simulink model "connect_pend_add"  (R2019b)
settings: Solver=VariableStepAuto  StartTime=0.0  StopTime=10.0  RelTol=1e-3
values from neighbouring files (symbols this model uses):
  Bd = 50    [anujay_single_pendulum_same.m]    (also in connect_pend_runner.m; double_pend_setup.m = [50,0;0,50])
  dampener = 100    [anujay_single_pendulum_same.m]    (also in connect_pend.m; connect_pend_runner.m; double_pend_setup.m = [50, 0; 0, 50])
  Dm1 = 30    [anujay_single_pendulum_same.m]    (also in connect_pend.m; connect_pend_runner.m; double_pend_setup.m = [30,0;0,30])
  g = 9.81    [G.m]    (also in connect_pend_runner.m = -9.81; run.m; single_pend_runner.m = -9.81)
  Kd = 50    [anujay_single_pendulum_same.m]    (also in connect_pend_runner.m; double_pend_setup.m = [50,0;0,50]; run.m = 300; single_pend_runner.m = 500)
  Km1 = 30    [anujay_single_pendulum_same.m]    (also in connect_pend.m; connect_pend_runner.m; double_pend_setup.m = [30, 0; 0 30])
  l1 = 1.0    (= 1)    [connect_pend.m]    (also in connect_pend_runner.m)
  l2 = l1    (= 1)    [connect_pend_runner.m]    (also in single_pend_runner.m = 3)
  lambda = 50.0    (= 50)    [connect_pend_runner.m]    (also in single_pend_runner.m = 1)
  lambda2 = 1.2    [anujay_single_pendulum_same.m]    (also in connect_pend_runner.m = 2.8; double_pend_setup.m = [5.0, 0; 0 5.0])
  m1 = 1.0    (= 1)    [connect_pend.m]    (also in connect_pend_runner.m)
  m2 = 1.0 + m1    (= 2)    [connect_pend.m]    (also in connect_pend_runner.m; single_pend_runner.m = 10)
  Md = 10    [anujay_single_pendulum_same.m]    (also in connect_pend_runner.m; double_pend_setup.m = [10, 0; 0, 20])
  rho = .50    (= 0.5)    [connect_pend_runner.m]
  rho2 = 100    [anujay_single_pendulum_same.m]    (also in connect_pend_runner.m = 4.5; double_pend_setup.m = [18, 0; 0, 18])
  spring = 100    [anujay_single_pendulum_same.m]    (also in connect_pend.m; connect_pend_runner.m; double_pend_setup.m = [50, 0; 0, 50])
libraries: robotcorelib x3, simulink x2
settings Model: Creator=nathanielgoldfarb  LastModifiedBy=nathanielgoldfarb
settings SolverCC: ZeroCrossAlgorithm=Adaptive
settings DebuggingCC: IgnoredZcDiagnostic=none

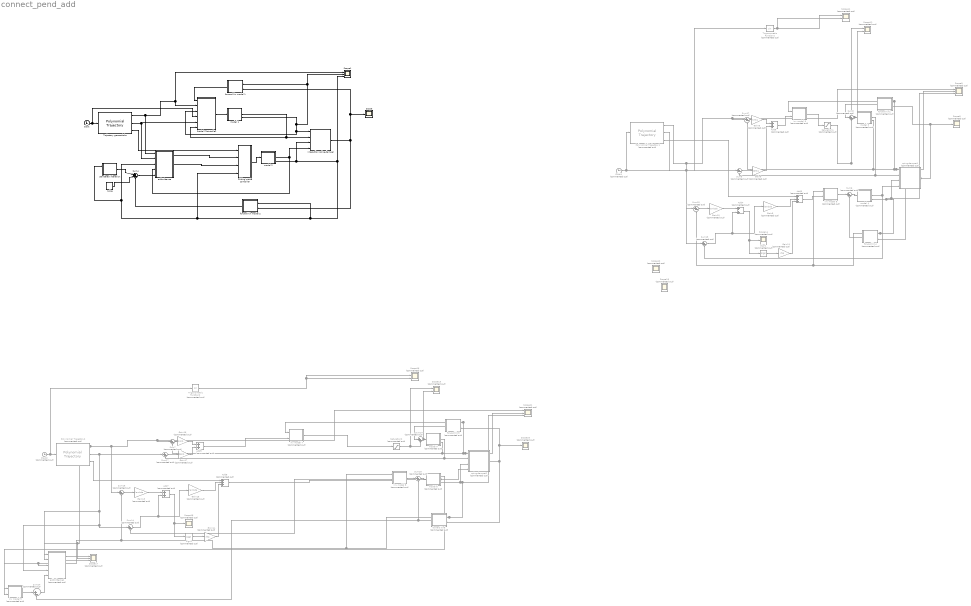
== system connect_pend_add ==
  " interaction sping-damper" : Subsystem
  Add{4,6..7,9} (4 alike) : Sum  Commented=on
  Add5 : Sum  Commented=on  Inputs=+++
  Add8 : Sum  Commented=on  Inputs=+++
  Clock : Clock
  Clock1 : Clock  Commented=on
  Clock2 : Clock  Commented=on
  Gain{5,10,13,15} (4 alike) : Gain  Commented=on  Gain=lambda
  Gain11 : Gain  Commented=on  Gain=rho
  Gain14 : Gain  Commented=on  Gain=rho
  Gain16 : Gain  Commented=on  Gain=Km1
  Gain17 : Gain  Commented=on  Gain=Dm1
  Gain8 : Gain  Commented=on  Gain=Km1
  Gain9 : Gain  Commented=on  Gain=Dm1
  Polynomial Trajectory1 : robotcorelib/Polynomial Trajectory  Commented=on  WaypointSource=Internal  Waypoints=[ -pi , 0 ]  TimePoints=[ 0, 3]  TimeInterval=[ 1, 4 ]  Method=Cubic Polynomial  ParameterSource=Internal  VelocityBoundaryCondition=zeros( 1, 2 )  AccelerationBoundaryCondition=zeros( 2, 5 )  SimulateUsing=Interpreted execution
      settings: SourceProductName=Robotics System Toolbox  SourceProductBaseCode=RO
  Polynomial Trajectory2 : robotcorelib/Polynomial Trajectory  Commented=on  WaypointSource=Internal  Waypoints=[ -pi , 0 ]  TimePoints=[ 0, 3]  TimeInterval=[ 1, 4 ]  Method=Cubic Polynomial  ParameterSource=Internal  VelocityBoundaryCondition=zeros( 1, 2 )  AccelerationBoundaryCondition=zeros( 2, 5 )  SimulateUsing=Interpreted execution
      settings: SourceProductName=Robotics System Toolbox  SourceProductBaseCode=RO
  Saturation1 : Saturate  Commented=on  UpperLimit=1.0  LowerLimit=-1.0
  Saturation2 : Saturate  Commented=on  UpperLimit=1.0  LowerLimit=-1.0
  Scope : Scope
  Scope1 : Scope  NumInputPorts=3
  Scope{10..13,15..16} (6 alike) : Scope  Commented=on  NumInputPorts=2
  Scope{8,14,18,20} (4 alike) : Scope  Commented=on
  Scope17 : Scope  Commented=on  NumInputPorts=3
  Scope21 : Scope  Commented=on  NumInputPorts=3
  Scope9 : Scope  Commented=on  NumInputPorts=3
  Sign1 : Signum  Commented=on
  Sign2 : Signum  Commented=on
  Sum{5..7,12..18,20} (11 alike) : Sum  Commented=on  Inputs=|+-
  Sum19 : Sum  Commented=on  Inputs=|++
  Sum4 : Sum  Inputs=|++-
  Sum8 : Sum  Commented=on  Inputs=|++
  Trajectory generatiobn : robotcorelib/Polynomial Trajectory  WaypointSource=Internal  Waypoints=[ -pi , 0 ]  TimePoints=[ 0, 3]  TimeInterval=[ 1, 4 ]  Method=Cubic Polynomial  ParameterSource=Internal  VelocityBoundaryCondition=zeros( 1, 2 )  AccelerationBoundaryCondition=zeros( 2, 5 )  SimulateUsing=Interpreted execution
      settings: SourceProductName=Robotics System Toolbox  SourceProductBaseCode=RO
  Trigonometric Function1 : Trigonometry  Commented=on
  Trigonometric Function2 : Trigonometry  Commented=on
  addmittacne1 : Subsystem  Commented=on
  addmittance : Subsystem
  forward kin model 1 : Subsystem
  forward kin model 2 : Subsystem
  forward kin1 : Subsystem  Commented=on
  forward kin4 : Subsystem  Commented=on
  forward kin5 : Subsystem  Commented=on
  forward kin6 : Subsystem  Commented=on
  inv model 5 : Subsystem  Commented=on
  inv model 6 : Subsystem  Commented=on
  inv model 7 : Subsystem  Commented=on
  inv model 8 : Subsystem  Commented=on
  inv model 9 : Subsystem  Commented=on
  model 1 : Subsystem
  model 1 controller : Subsystem
  model 2 : Subsystem
  model 3 : Subsystem  Commented=on
  model 4 : Subsystem  Commented=on
  model 5 : Subsystem  Commented=on
  model 6 : Subsystem  Commented=on
  noise : UniformRandomNumber  Minimum=-3  Maximum=3  SampleTime=0.1
  sliding mode controller : Subsystem
  sping-damper1 : Subsystem  Commented=on
  sping-damper2 : Subsystem  Commented=on
  standered interation : Subsystem
  wires:
  model 1/3(pos) -> model 1 controller/3(q), " interaction sping-damper"/1(theta 1), Scope1/2, forward kin model 1/1("theta ")  "model 1"
  " interaction sping-damper"/1(F) -> Scope/1, forward kin model 1/2(F), forward kin model 2/2(F)
  model 2/3(pos) -> forward kin model 2/1("theta "), addmittance/3(q), standered interation/1(q), sliding mode controller/4(q), Scope1/3, " interaction sping-damper"/3(theta 2)  "model 2"
  model 2/2(vel) -> addmittance/4(qd), " interaction sping-damper"/4(dtheta 2)  "model 2"
  forward kin model 2/1("tau ") -> Sum4/3  "Ti"
  Sum4/1 -> addmittance/5(force)
  standered interation/1("tau ") -> Sum4/1  "Tid"
  model 4/3(pos) -> Scope9/3, sping-damper1/3(theta 2), Sum15/2, inv model 6/1(q), forward kin4/1("theta ")  "model 2"
  sping-damper1/1(F) -> Scope8/1, forward kin1/2(F), forward kin4/2(F)
  Add6/1 -> inv model 5/2("u ")
  Clock1/1 -> Trigonometric Function1/1, Polynomial Trajectory1/1
  model 3/3(pos) -> forward kin1/1("theta "), inv model 5/1(q), Scope9/2, sping-damper1/1(theta 1), Sum12/2  "model 1"
  Gain11/1 -> Add5/3
  Gain10/1 -> Add4/1
  forward kin1/1("tau ") -> Sum8/1
  Add5/1 -> inv model 6/2("u ")
  Gain9/1 -> Add6/2
  Saturation1/1 -> Scope10/1, Sum8/2
  model 4/2(vel) -> sping-damper1/4(dtheta 2), Sum13/2  "model 2"
  Sum12/1 -> Gain8/1
  Sign1/1 -> Gain11/1
  Trigonometric Function1/1 -> Scope11/1, Scope11/2
  inv model 5/1("tau ") -> Saturation1/1
  model 3/2(vel) -> sping-damper1/2(dtheta 1), Sum5/2
  Gain8/1 -> Add6/1
  Sum8/1 -> Scope10/2, model 3/1("u ")
  Sum5/1 -> Gain9/1
  Add4/1 -> Sign1/1, Scope14/1
  Polynomial Trajectory1/2 -> Sum5/1, Sum13/1
  Polynomial Trajectory1/1 -> Scope9/1, Sum12/1, Sum15/1
  Sum15/1 -> Gain10/1
  Sum13/1 -> Gain5/1, Add4/2
  Polynomial Trajectory1/3 -> Add5/1
  inv model 6/1("tau ") -> Sum6/1  "SMC"
  Sum6/1 -> model 4/1("u ")
  Gain5/1 -> Add5/2
  forward kin4/1("tau ") -> Sum6/2
  Gain13/1 -> Add7/1
  Gain14/1 -> Add8/3
  Gain17/1 -> Add9/2
  Add8/1 -> inv model 8/2("u ")
  Sum14/1 -> Gain15/1, Add7/2
  model 5/2(vel) -> sping-damper2/2(dtheta 1), Sum17/2
  Sum17/1 -> Gain17/1
  Add9/1 -> inv model 7/2("u ")
  Sign2/1 -> Gain14/1
  Clock2/1 -> Trigonometric Function2/1, Polynomial Trajectory2/1
  sping-damper2/1(F) -> forward kin6/2(F), Scope20/1, forward kin5/2(F)
  Sum19/1 -> Scope13/2, model 5/1("u ")
  Gain15/1 -> Add8/2
  Saturation2/1 -> Scope13/1, Sum19/2
  Polynomial Trajectory2/1 -> Scope21/1, Sum7/1, Sum16/1, addmittacne1/1(q desird), Scope17/2
  inv model 8/1("tau ") -> Sum18/1  "SMC"
  Sum7/1 -> Gain16/1
  forward kin6/1("tau ") -> Sum20/2, Sum18/2
  model 6/3(pos) -> Scope21/3, inv model 9/1(q), addmittacne1/3(q), Scope17/3, Sum16/2, inv model 8/1(q), forward kin6/1("theta "), sping-damper2/3(theta 2)  "model 2"
  Polynomial Trajectory2/3 -> Add8/1
  forward kin5/1("tau ") -> Sum19/1
  model 5/3(pos) -> forward kin5/1("theta "), inv model 7/1(q), Scope21/2, sping-damper2/1(theta 1), Sum7/2  "model 1"
  Sum16/1 -> Gain13/1
  Polynomial Trajectory2/2 -> Sum17/1, addmittacne1/2(qd desird), Sum14/1, addmittacne1/4(qd)
  model 6/2(vel) -> sping-damper2/4(dtheta 2), Sum14/2  "model 2"
  inv model 7/1("tau ") -> Saturation2/1
  Sum18/1 -> model 6/1("u ")
  Gain16/1 -> Add9/1
  Add7/1 -> Sign2/1, Scope18/1
  Trigonometric Function2/1 -> Scope16/1, Scope16/2
  inv model 9/1("tau ") -> Sum20/1  "SMC"
  Sum20/1 -> addmittacne1/5(force)
  model 6/1(accel) -> inv model 9/2("u ")
  addmittacne1/1(q_add) -> Scope17/1
  noise/1 -> Sum4/2
  addmittance/1(q_add) -> sliding mode controller/2(x)  "x"
  model 1/2(vel) -> model 1 controller/6(qd), " interaction sping-damper"/2(dtheta 1)
  Trajectory generatiobn/2 -> model 1 controller/5(qd desired), addmittance/2(qd desird)
  Trajectory generatiobn/1 -> addmittance/1(q desird), model 1 controller/2(q desired), Scope1/1
  Clock/1 -> model 1 controller/4(t), Trajectory generatiobn/1
  forward kin model 1/1("tau ") -> model 1 controller/1(interaction torque)
  model 1 controller/1(u) -> model 1/1("u ")
  Trajectory generatiobn/3 -> sliding mode controller/1(qdd desired)
  addmittance/2(qd_add) -> sliding mode controller/3(xd)  "xd"
  sliding mode controller/1(SMC) -> model 2/1("u ")

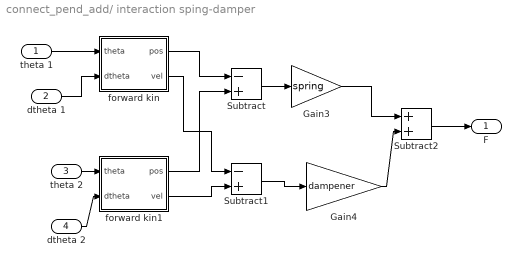
== system connect_pend_add/ interaction sping-damper ==
  theta 1 : Inport
  dtheta 1 : Inport  Port=2
  theta 2 : Inport  Port=3
  dtheta 2 : Inport  Port=4
  Gain3 : Gain  Gain=spring
  Gain4 : Gain  Gain=dampener
  Subtract : Sum  Inputs=-+
  Subtract1 : Sum  Inputs=-+
  Subtract2 : Sum
  forward kin : Subsystem
  forward kin1 : Subsystem
  F : Outport
  wires:
  Subtract2/1 -> F/1
  forward kin/2(vel) -> Subtract1/1
  Gain4/1 -> Subtract2/2
  Subtract1/1 -> Gain4/1
  dtheta 1/1 -> forward kin/2("dtheta ")
  forward kin1/1(pos) -> Subtract/2
  theta 1/1 -> forward kin/1("theta ")
  Subtract/1 -> Gain3/1
  forward kin/1(pos) -> Subtract/1
  dtheta 2/1 -> forward kin1/2("dtheta ")
  theta 2/1 -> forward kin1/1("theta ")
  forward kin1/2(vel) -> Subtract1/2
  Gain3/1 -> Subtract2/1

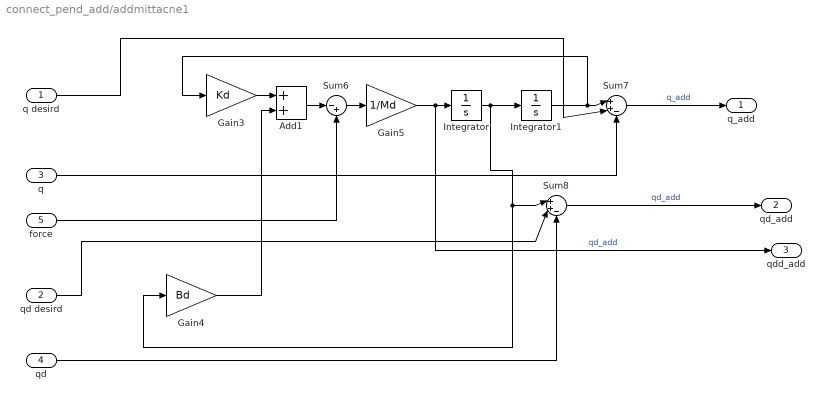
== system connect_pend_add/addmittacne1 ==
  q desird : Inport
  qd desird : Inport  Port=2
  q : Inport  Port=3
  qd : Inport  Port=4
  force : Inport  Port=5
  Add1 : Sum
  Gain3 : Gain  Gain=Kd
  Gain4 : Gain  Gain=Bd
  Gain5 : Gain  Gain=1/Md
  Integrator : Integrator
  Integrator1 : Integrator  InitialCondition=-3
  Sum6 : Sum  Inputs=|-+
  Sum7 : Sum  Inputs=|++-
  Sum8 : Sum  Inputs=|++-
  q_add : Outport
  qd_add : Outport  Port=2
  qdd_add : Outport  Port=3
  wires:
  Sum6/1 -> Gain5/1
  Integrator1/1 -> Gain3/1, Sum7/1
  Integrator/1 -> Gain4/1, Sum8/1, Integrator1/1
  q desird/1 -> Sum7/2
  Gain3/1 -> Add1/1
  Gain4/1 -> Add1/2
  force/1 -> Sum6/2
  qd desird/1 -> Sum8/2
  Sum8/1 -> qd_add/1  "qd_add"
  Add1/1 -> Sum6/1
  Sum7/1 -> q_add/1  "q_add"
  Gain5/1 -> qdd_add/1, Integrator/1  "qd_add"
  qd/1 -> Sum8/3
  q/1 -> Sum7/3

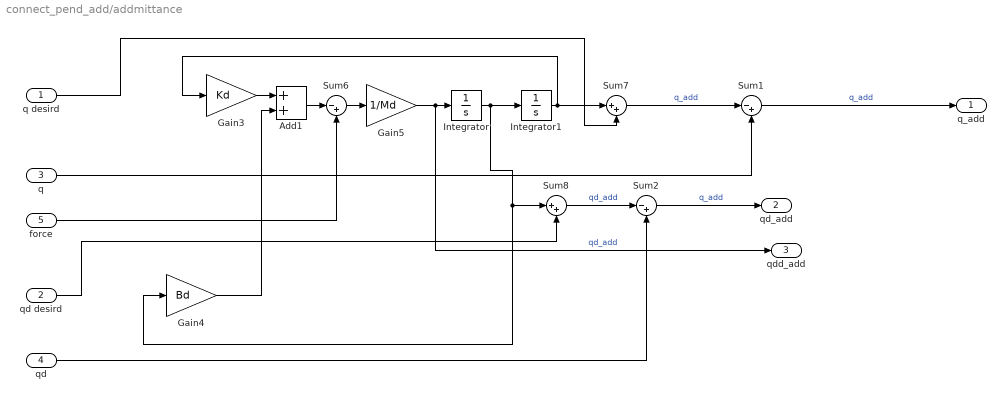
== system connect_pend_add/addmittance ==
  q desird : Inport
  qd desird : Inport  Port=2
  q : Inport  Port=3
  qd : Inport  Port=4
  force : Inport  Port=5
  Add1 : Sum
  Gain3 : Gain  Gain=Kd
  Gain4 : Gain  Gain=Bd
  Gain5 : Gain  Gain=1/Md
  Integrator : Integrator
  Integrator1 : Integrator  InitialCondition=pi
  Sum1 : Sum  Inputs=|-+
  Sum2 : Sum  Inputs=|-+
  Sum6 : Sum  Inputs=|-+
  Sum7 : Sum  Inputs=|++
  Sum8 : Sum  Inputs=|++
  q_add : Outport
  qd_add : Outport  Port=2
  qdd_add : Outport  Port=3
  wires:
  Sum7/1 -> Sum1/1  "q_add"
  Add1/1 -> Sum6/1
  force/1 -> Sum6/2
  qd desird/1 -> Sum8/2
  Gain5/1 -> qdd_add/1, Integrator/1  "qd_add"
  Sum6/1 -> Gain5/1
  Gain4/1 -> Add1/2
  Gain3/1 -> Add1/1
  Integrator/1 -> Gain4/1, Sum8/1, Integrator1/1
  q desird/1 -> Sum7/2
  Sum8/1 -> Sum2/1  "qd_add"
  Integrator1/1 -> Gain3/1, Sum7/1
  qd/1 -> Sum2/2
  Sum1/1 -> q_add/1  "q_add"
  q/1 -> Sum1/2
  Sum2/1 -> qd_add/1  "q_add"

== system connect_pend_add/forward kin model 1 ==
  "theta " : Inport
  F : Inport  Port=2
  Gain3 : Gain  Gain=-l1
  Gain4 : Gain  Gain=l1
  Mux : Mux  Inputs=2
  Product : Product  Multiplication=Matrix(*)
  Transpose : Math  Operator=transpose  SignedPower=off  SaturateOnIntegerOverflow=on
  Trigonometric Function : Trigonometry
  Trigonometric Function1 : Trigonometry  Operator=cos
  XY Graph : simulink/Sinks/XY Graph  xmin=-1  xmax=1  ymin=-1  ymax=1  st=-1
  "tau " : Outport
  wires:
  "theta "/1 -> Trigonometric Function1/1, Trigonometric Function/1
  Gain4/1 -> XY Graph/2, Mux/2
  Trigonometric Function/1 -> Gain3/1
  Gain3/1 -> XY Graph/1, Mux/1
  Trigonometric Function1/1 -> Gain4/1
  Mux/1 -> Transpose/1
  Transpose/1 -> Product/1
  F/1 -> Product/2
  Product/1 -> "tau "/1

== system connect_pend_add/forward kin model 2 ==
  "theta " : Inport
  F : Inport  Port=2
  Gain3 : Gain  Gain=-l1
  Gain4 : Gain  Gain=l1
  Mux : Mux  Inputs=2
  Product : Product  Multiplication=Matrix(*)
  Transpose : Math  Operator=transpose  SignedPower=off  SaturateOnIntegerOverflow=on
  Trigonometric Function : Trigonometry
  Trigonometric Function1 : Trigonometry  Operator=cos
  "tau " : Outport
  wires:
  "theta "/1 -> Trigonometric Function1/1, Trigonometric Function/1
  Gain4/1 -> Mux/2
  Trigonometric Function/1 -> Gain3/1
  Gain3/1 -> Mux/1
  Trigonometric Function1/1 -> Gain4/1
  Mux/1 -> Transpose/1
  Transpose/1 -> Product/1
  F/1 -> Product/2
  Product/1 -> "tau "/1

== system connect_pend_add/forward kin1 ==
  "theta " : Inport
  F : Inport  Port=2
  Gain3 : Gain  Gain=-l1
  Gain4 : Gain  Gain=l1
  Mux : Mux  Inputs=2
  Product : Product  Multiplication=Matrix(*)
  Transpose : Math  Operator=transpose  SignedPower=off  SaturateOnIntegerOverflow=on
  Trigonometric Function : Trigonometry
  Trigonometric Function1 : Trigonometry  Operator=cos
  "tau " : Outport
  wires:
  "theta "/1 -> Trigonometric Function1/1, Trigonometric Function/1
  Gain4/1 -> Mux/2
  Trigonometric Function/1 -> Gain3/1
  Gain3/1 -> Mux/1
  Trigonometric Function1/1 -> Gain4/1
  Mux/1 -> Transpose/1
  Transpose/1 -> Product/1
  F/1 -> Product/2
  Product/1 -> "tau "/1

== system connect_pend_add/forward kin4 ==
  "theta " : Inport
  F : Inport  Port=2
  Gain3 : Gain  Gain=-l1
  Gain4 : Gain  Gain=l1
  Mux : Mux  Inputs=2
  Product : Product  Multiplication=Matrix(*)
  Transpose : Math  Operator=transpose  SignedPower=off  SaturateOnIntegerOverflow=on
  Trigonometric Function : Trigonometry
  Trigonometric Function1 : Trigonometry  Operator=cos
  "tau " : Outport
  wires:
  "theta "/1 -> Trigonometric Function1/1, Trigonometric Function/1
  Gain4/1 -> Mux/2
  Trigonometric Function/1 -> Gain3/1
  Gain3/1 -> Mux/1
  Trigonometric Function1/1 -> Gain4/1
  Mux/1 -> Transpose/1
  Transpose/1 -> Product/1
  F/1 -> Product/2
  Product/1 -> "tau "/1

== system connect_pend_add/forward kin5 ==
  "theta " : Inport
  F : Inport  Port=2
  Gain3 : Gain  Gain=-l1
  Gain4 : Gain  Gain=l1
  Mux : Mux  Inputs=2
  Product : Product  Multiplication=Matrix(*)
  Transpose : Math  Operator=transpose  SignedPower=off  SaturateOnIntegerOverflow=on
  Trigonometric Function : Trigonometry
  Trigonometric Function1 : Trigonometry  Operator=cos
  "tau " : Outport
  wires:
  "theta "/1 -> Trigonometric Function1/1, Trigonometric Function/1
  Gain4/1 -> Mux/2
  Trigonometric Function/1 -> Gain3/1
  Gain3/1 -> Mux/1
  Trigonometric Function1/1 -> Gain4/1
  Mux/1 -> Transpose/1
  Transpose/1 -> Product/1
  F/1 -> Product/2
  Product/1 -> "tau "/1

== system connect_pend_add/forward kin6 ==
  "theta " : Inport
  F : Inport  Port=2
  Gain3 : Gain  Gain=-l1
  Gain4 : Gain  Gain=l1
  Mux : Mux  Inputs=2
  Product : Product  Multiplication=Matrix(*)
  Transpose : Math  Operator=transpose  SignedPower=off  SaturateOnIntegerOverflow=on
  Trigonometric Function : Trigonometry
  Trigonometric Function1 : Trigonometry  Operator=cos
  "tau " : Outport
  wires:
  "theta "/1 -> Trigonometric Function1/1, Trigonometric Function/1
  Gain4/1 -> Mux/2
  Trigonometric Function/1 -> Gain3/1
  Gain3/1 -> Mux/1
  Trigonometric Function1/1 -> Gain4/1
  Mux/1 -> Transpose/1
  Transpose/1 -> Product/1
  F/1 -> Product/2
  Product/1 -> "tau "/1

== system connect_pend_add/inv model 5 ==
  q : Inport
  "u " : Inport  Port=2
  Add1 : Sum
  Constant1 : Constant  Value=m1*g*l1
  Gain3 : Gain  Gain=m1*l1*l1
  Product1 : Product
  Trigonometric Function1 : Trigonometry
  "tau " : Outport
  wires:
  Product1/1 -> Add1/1
  Constant1/1 -> Product1/2
  Add1/1 -> "tau "/1
  Gain3/1 -> Add1/2
  "u "/1 -> Gain3/1
  Trigonometric Function1/1 -> Product1/1
  q/1 -> Trigonometric Function1/1

== system connect_pend_add/inv model 6 ==
  q : Inport
  "u " : Inport  Port=2
  Add1 : Sum
  Constant1 : Constant  Value=m2*g*l2
  Gain3 : Gain  Gain=m2*l2*l2
  Product1 : Product
  Trigonometric Function1 : Trigonometry
  "tau " : Outport
  wires:
  Product1/1 -> Add1/1
  Constant1/1 -> Product1/2
  Add1/1 -> "tau "/1
  Gain3/1 -> Add1/2
  "u "/1 -> Gain3/1
  Trigonometric Function1/1 -> Product1/1
  q/1 -> Trigonometric Function1/1

== system connect_pend_add/inv model 7 ==
  q : Inport
  "u " : Inport  Port=2
  Add1 : Sum
  Constant1 : Constant  Value=m1*g*l1
  Gain3 : Gain  Gain=m1*l1*l1
  Product1 : Product
  Trigonometric Function1 : Trigonometry
  "tau " : Outport
  wires:
  Product1/1 -> Add1/1
  Constant1/1 -> Product1/2
  Add1/1 -> "tau "/1
  Gain3/1 -> Add1/2
  "u "/1 -> Gain3/1
  Trigonometric Function1/1 -> Product1/1
  q/1 -> Trigonometric Function1/1

== system connect_pend_add/inv model 8 ==
  q : Inport
  "u " : Inport  Port=2
  Add1 : Sum
  Constant1 : Constant  Value=m2*g*l2
  Gain3 : Gain  Gain=m2*l2*l2
  Product1 : Product
  Trigonometric Function1 : Trigonometry
  "tau " : Outport
  wires:
  Product1/1 -> Add1/1
  Constant1/1 -> Product1/2
  Add1/1 -> "tau "/1
  Gain3/1 -> Add1/2
  "u "/1 -> Gain3/1
  Trigonometric Function1/1 -> Product1/1
  q/1 -> Trigonometric Function1/1

== system connect_pend_add/inv model 9 ==
  q : Inport
  "u " : Inport  Port=2
  Add1 : Sum
  Constant1 : Constant  Value=m2*g*l2
  Gain3 : Gain  Gain=m2*l2*l2
  Product1 : Product
  Trigonometric Function1 : Trigonometry
  "tau " : Outport
  wires:
  Product1/1 -> Add1/1
  Constant1/1 -> Product1/2
  Add1/1 -> "tau "/1
  Gain3/1 -> Add1/2
  "u "/1 -> Gain3/1
  Trigonometric Function1/1 -> Product1/1
  q/1 -> Trigonometric Function1/1

== system connect_pend_add/model 1 ==
  "u " : Inport
  Add : Sum  Inputs=+-
  Constant : Constant  Value=m1*g*l1
  Gain : Gain  Gain=1/(m1*l1*l1)
  Integrator : Integrator
  Integrator1 : Integrator  InitialCondition=-pi
  Product : Product
  Trigonometric Function : Trigonometry
  accel : Outport
  vel : Outport  Port=2
  pos : Outport  Port=3
  wires:
  Integrator1/1 -> pos/1, Trigonometric Function/1
  "u "/1 -> Add/1
  Constant/1 -> Product/2
  Add/1 -> Gain/1
  Trigonometric Function/1 -> Product/1
  Product/1 -> Add/2
  Gain/1 -> accel/1, Integrator/1
  Integrator/1 -> vel/1, Integrator1/1

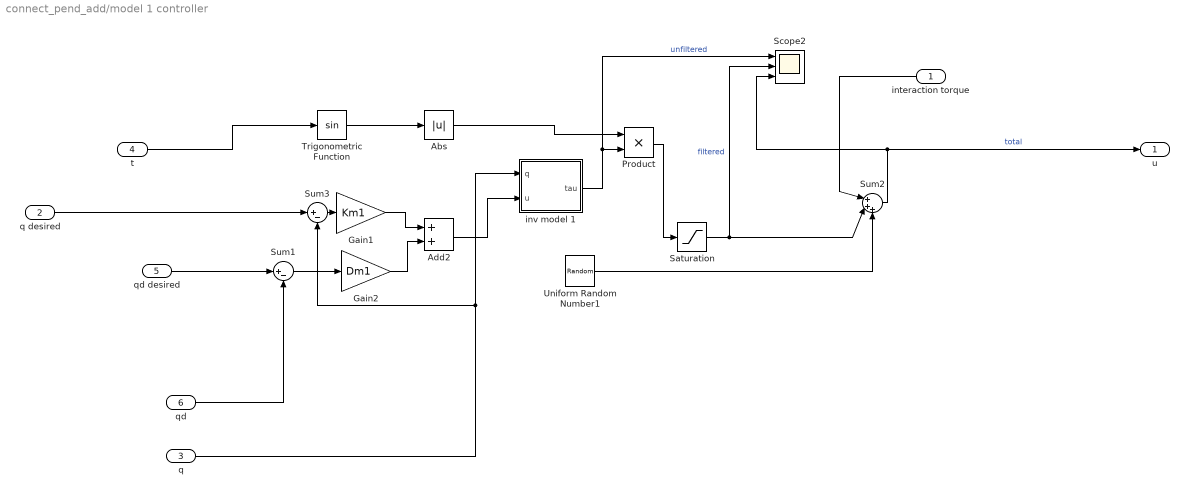
== system connect_pend_add/model 1 controller ==
  interaction torque : Inport
  q desired : Inport  Port=2
  q : Inport  Port=3
  t : Inport  Port=4
  qd desired : Inport  Port=5
  qd : Inport  Port=6
  Abs : Abs
  Add2 : Sum
  Gain1 : Gain  Gain=Km1
  Gain2 : Gain  Gain=Dm1
  Product : Product
  Saturation : Saturate
  Scope2 : Scope  NumInputPorts=3
  Sum1 : Sum  Inputs=|+-
  Sum2 : Sum  Inputs=|+++
  Sum3 : Sum  Inputs=|+-
  Trigonometric Function : Trigonometry
  Uniform Random Number1 : UniformRandomNumber  Minimum=-4  Maximum=4  SampleTime=0.1
  inv model 1 : Subsystem
  u : Outport
  wires:
  Sum1/1 -> Gain2/1
  Product/1 -> Saturation/1
  qd/1 -> Sum1/2
  Uniform Random Number1/1 -> Sum2/3
  Sum2/1 -> u/1, Scope2/3  "total"
  Sum3/1 -> Gain1/1
  Gain2/1 -> Add2/2
  Abs/1 -> Product/1
  interaction torque/1 -> Sum2/1
  q desired/1 -> Sum3/1
  Add2/1 -> inv model 1/2("u ")
  Gain1/1 -> Add2/1
  inv model 1/1("tau ") -> Scope2/1, Product/2  "unfiltered"
  t/1 -> Trigonometric Function/1
  qd desired/1 -> Sum1/1
  q/1 -> Sum3/2, inv model 1/1(q)
  Trigonometric Function/1 -> Abs/1
  Saturation/1 -> Scope2/2, Sum2/2  "filtered"

== system connect_pend_add/model 2 ==
  "u " : Inport
  Add : Sum  Inputs=+-
  Constant : Constant  Value=m2*g*l2
  Gain : Gain  Gain=1/(m2*l2*l2)
  Integrator : Integrator
  Integrator1 : Integrator  InitialCondition=-pi
  Product : Product
  Trigonometric Function : Trigonometry
  accel : Outport
  vel : Outport  Port=2
  pos : Outport  Port=3
  wires:
  Integrator1/1 -> pos/1, Trigonometric Function/1
  "u "/1 -> Add/1
  Constant/1 -> Product/2
  Add/1 -> Gain/1
  Trigonometric Function/1 -> Product/1
  Product/1 -> Add/2
  Gain/1 -> accel/1, Integrator/1
  Integrator/1 -> vel/1, Integrator1/1

== system connect_pend_add/model 3 ==
  "u " : Inport
  Add : Sum  Inputs=+-
  Constant : Constant  Value=m1*g*l1
  Gain : Gain  Gain=1/(m1*l1*l1)
  Integrator : Integrator
  Integrator1 : Integrator  InitialCondition=-pi
  Product : Product
  Trigonometric Function : Trigonometry
  accel : Outport
  vel : Outport  Port=2
  pos : Outport  Port=3
  wires:
  Integrator1/1 -> pos/1, Trigonometric Function/1
  "u "/1 -> Add/1
  Constant/1 -> Product/2
  Add/1 -> Gain/1
  Trigonometric Function/1 -> Product/1
  Product/1 -> Add/2
  Gain/1 -> accel/1, Integrator/1
  Integrator/1 -> vel/1, Integrator1/1

== system connect_pend_add/model 4 ==
  "u " : Inport
  Add : Sum  Inputs=+-
  Constant : Constant  Value=m2*g*l2
  Gain : Gain  Gain=1/(m2*l2*l2)
  Integrator : Integrator
  Integrator1 : Integrator  InitialCondition=-pi
  Product : Product
  Trigonometric Function : Trigonometry
  accel : Outport
  vel : Outport  Port=2
  pos : Outport  Port=3
  wires:
  Integrator1/1 -> pos/1, Trigonometric Function/1
  "u "/1 -> Add/1
  Constant/1 -> Product/2
  Add/1 -> Gain/1
  Trigonometric Function/1 -> Product/1
  Product/1 -> Add/2
  Gain/1 -> accel/1, Integrator/1
  Integrator/1 -> vel/1, Integrator1/1

== system connect_pend_add/model 5 ==
  "u " : Inport
  Add : Sum  Inputs=+-
  Constant : Constant  Value=m1*g*l1
  Gain : Gain  Gain=1/(m1*l1*l1)
  Integrator : Integrator
  Integrator1 : Integrator  InitialCondition=-pi
  Product : Product
  Trigonometric Function : Trigonometry
  accel : Outport
  vel : Outport  Port=2
  pos : Outport  Port=3
  wires:
  Integrator1/1 -> pos/1, Trigonometric Function/1
  "u "/1 -> Add/1
  Constant/1 -> Product/2
  Add/1 -> Gain/1
  Trigonometric Function/1 -> Product/1
  Product/1 -> Add/2
  Gain/1 -> accel/1, Integrator/1
  Integrator/1 -> vel/1, Integrator1/1

== system connect_pend_add/model 6 ==
  "u " : Inport
  Add : Sum  Inputs=+-
  Constant : Constant  Value=m2*g*l2
  Gain : Gain  Gain=1/(m2*l2*l2)
  Integrator : Integrator
  Integrator1 : Integrator  InitialCondition=-pi
  Product : Product
  Trigonometric Function : Trigonometry
  accel : Outport
  vel : Outport  Port=2
  pos : Outport  Port=3
  wires:
  Integrator1/1 -> pos/1, Trigonometric Function/1
  "u "/1 -> Add/1
  Constant/1 -> Product/2
  Add/1 -> Gain/1
  Trigonometric Function/1 -> Product/1
  Product/1 -> Add/2
  Gain/1 -> accel/1, Integrator/1
  Integrator/1 -> vel/1, Integrator1/1

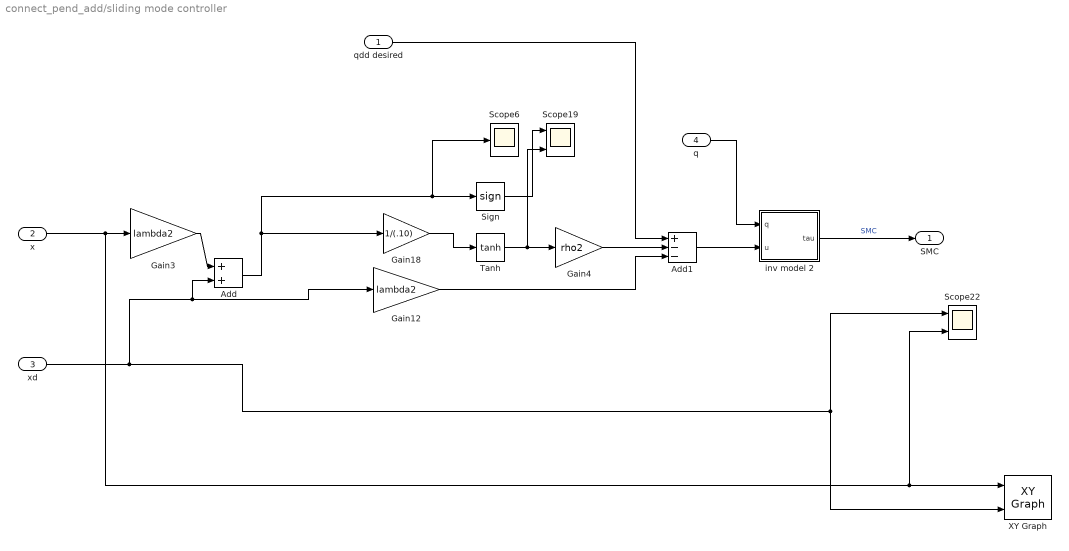
== system connect_pend_add/sliding mode controller ==
  qdd desired : Inport
  x : Inport  Port=2
  xd : Inport  Port=3
  q : Inport  Port=4
  Add : Sum
  Add1 : Sum  Inputs=+--
  Gain12 : Gain  Gain=lambda2
  Gain18 : Gain  Gain=1/(.10)
  Gain3 : Gain  Gain=lambda2
  Gain4 : Gain  Gain=rho2
  Scope19 : Scope  NumInputPorts=2
  Scope22 : Scope  NumInputPorts=2
  Scope6 : Scope
  Sign : Signum
  Tanh : Trigonometry  Operator=tanh
  XY Graph : simulink/Sinks/XY Graph  xmin=-5  xmax=2  ymin=0  ymax=3  st=0.01
  inv model 2 : Subsystem
  SMC : Outport
  wires:
  Gain18/1 -> Tanh/1
  Gain12/1 -> Add1/3
  Gain3/1 -> Add/1
  inv model 2/1("tau ") -> SMC/1  "SMC"
  q/1 -> inv model 2/1(q)
  x/1 -> Scope22/2, XY Graph/1, Gain3/1
  xd/1 -> Add/2, Gain12/1, XY Graph/2, Scope22/1
  Add/1 -> Gain18/1, Scope6/1, Sign/1
  Add1/1 -> inv model 2/2("u ")
  Sign/1 -> Scope19/1
  Gain4/1 -> Add1/2
  qdd desired/1 -> Add1/1
  Tanh/1 -> Scope19/2, Gain4/1

== system connect_pend_add/sping-damper1 ==
  theta 1 : Inport
  dtheta 1 : Inport  Port=2
  theta 2 : Inport  Port=3
  dtheta 2 : Inport  Port=4
  Gain3 : Gain  Gain=spring
  Gain4 : Gain  Gain=dampener
  Subtract : Sum  Inputs=-+
  Subtract1 : Sum  Inputs=-+
  Subtract2 : Sum
  forward kin : Subsystem
  forward kin1 : Subsystem
  F : Outport
  wires:
  Subtract2/1 -> F/1
  forward kin/2(vel) -> Subtract1/1
  Gain4/1 -> Subtract2/2
  Subtract1/1 -> Gain4/1
  dtheta 1/1 -> forward kin/2("dtheta ")
  forward kin1/1(pos) -> Subtract/2
  theta 1/1 -> forward kin/1("theta ")
  Subtract/1 -> Gain3/1
  forward kin/1(pos) -> Subtract/1
  dtheta 2/1 -> forward kin1/2("dtheta ")
  theta 2/1 -> forward kin1/1("theta ")
  forward kin1/2(vel) -> Subtract1/2
  Gain3/1 -> Subtract2/1

== system connect_pend_add/sping-damper2 ==
  theta 1 : Inport
  dtheta 1 : Inport  Port=2
  theta 2 : Inport  Port=3
  dtheta 2 : Inport  Port=4
  Gain3 : Gain  Gain=spring
  Gain4 : Gain  Gain=dampener
  Subtract : Sum  Inputs=-+
  Subtract1 : Sum  Inputs=-+
  Subtract2 : Sum
  forward kin : Subsystem
  forward kin1 : Subsystem
  F : Outport
  wires:
  Subtract2/1 -> F/1
  forward kin/2(vel) -> Subtract1/1
  Gain4/1 -> Subtract2/2
  Subtract1/1 -> Gain4/1
  dtheta 1/1 -> forward kin/2("dtheta ")
  forward kin1/1(pos) -> Subtract/2
  theta 1/1 -> forward kin/1("theta ")
  Subtract/1 -> Gain3/1
  forward kin/1(pos) -> Subtract/1
  dtheta 2/1 -> forward kin1/2("dtheta ")
  theta 2/1 -> forward kin1/1("theta ")
  forward kin1/2(vel) -> Subtract1/2
  Gain3/1 -> Subtract2/1

== system connect_pend_add/standered interation ==
  q : Inport
  "u " : Inport  Port=2
  Add1 : Sum
  Constant1 : Constant  Value=m1*g*l1
  Gain3 : Gain  Gain=m1*l1*l1
  Product1 : Product
  Trigonometric Function1 : Trigonometry
  "tau " : Outport
  wires:
  Product1/1 -> Add1/1
  Constant1/1 -> Product1/2
  Add1/1 -> "tau "/1
  Gain3/1 -> Add1/2
  "u "/1 -> Gain3/1
  Trigonometric Function1/1 -> Product1/1
  q/1 -> Trigonometric Function1/1

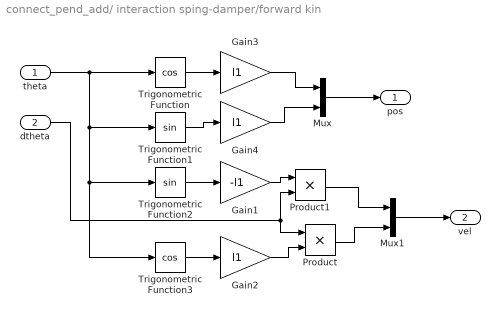
== system connect_pend_add/ interaction sping-damper/forward kin ==
  "theta " : Inport
  "dtheta " : Inport  Port=2
  Gain1 : Gain  Gain=-l1
  Gain2 : Gain  Gain=l1
  Gain3 : Gain  Gain=l1
  Gain4 : Gain  Gain=l1
  Mux : Mux  Inputs=2
  Mux1 : Mux  Inputs=2
  Product : Product
  Product1 : Product
  Trigonometric Function : Trigonometry  Operator=cos
  Trigonometric Function1 : Trigonometry
  Trigonometric Function2 : Trigonometry
  Trigonometric Function3 : Trigonometry  Operator=cos
  pos : Outport
  vel : Outport  Port=2
  wires:
  "theta "/1 -> Trigonometric Function3/1, Trigonometric Function2/1, Trigonometric Function1/1, Trigonometric Function/1
  Gain4/1 -> Mux/2
  Trigonometric Function/1 -> Gain3/1
  Gain3/1 -> Mux/1
  Trigonometric Function1/1 -> Gain4/1
  Trigonometric Function3/1 -> Gain2/1
  Trigonometric Function2/1 -> Gain1/1
  Gain1/1 -> Product1/1
  "dtheta "/1 -> Product1/2, Product/1
  Gain2/1 -> Product/2
  Product1/1 -> Mux1/1
  Product/1 -> Mux1/2
  Mux/1 -> pos/1
  Mux1/1 -> vel/1

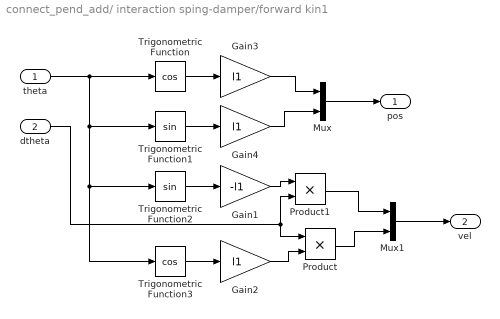
== system connect_pend_add/ interaction sping-damper/forward kin1 ==
  "theta " : Inport
  "dtheta " : Inport  Port=2
  Gain1 : Gain  Gain=-l1
  Gain2 : Gain  Gain=l1
  Gain3 : Gain  Gain=l1
  Gain4 : Gain  Gain=l1
  Mux : Mux  Inputs=2
  Mux1 : Mux  Inputs=2
  Product : Product
  Product1 : Product
  Trigonometric Function : Trigonometry  Operator=cos
  Trigonometric Function1 : Trigonometry
  Trigonometric Function2 : Trigonometry
  Trigonometric Function3 : Trigonometry  Operator=cos
  pos : Outport
  vel : Outport  Port=2
  wires:
  "theta "/1 -> Trigonometric Function3/1, Trigonometric Function2/1, Trigonometric Function1/1, Trigonometric Function/1
  Gain4/1 -> Mux/2
  Trigonometric Function/1 -> Gain3/1
  Gain3/1 -> Mux/1
  Trigonometric Function1/1 -> Gain4/1
  Trigonometric Function3/1 -> Gain2/1
  Trigonometric Function2/1 -> Gain1/1
  Gain1/1 -> Product1/1
  "dtheta "/1 -> Product1/2, Product/1
  Gain2/1 -> Product/2
  Product1/1 -> Mux1/1
  Product/1 -> Mux1/2
  Mux/1 -> pos/1
  Mux1/1 -> vel/1

== system connect_pend_add/model 1 controller/inv model 1 ==
  q : Inport
  "u " : Inport  Port=2
  Add1 : Sum
  Constant1 : Constant  Value=m1*g*l1
  Gain3 : Gain  Gain=m1*l1*l1
  Product1 : Product
  Trigonometric Function1 : Trigonometry
  "tau " : Outport
  wires:
  Product1/1 -> Add1/1
  Constant1/1 -> Product1/2
  Add1/1 -> "tau "/1
  Gain3/1 -> Add1/2
  "u "/1 -> Gain3/1
  Trigonometric Function1/1 -> Product1/1
  q/1 -> Trigonometric Function1/1

== system connect_pend_add/sliding mode controller/inv model 2 ==
  q : Inport
  "u " : Inport  Port=2
  Add1 : Sum
  Constant1 : Constant  Value=m2*g*l2
  Gain3 : Gain  Gain=m2*l2*l2
  Product1 : Product
  Trigonometric Function1 : Trigonometry
  "tau " : Outport
  wires:
  Product1/1 -> Add1/1
  Constant1/1 -> Product1/2
  Add1/1 -> "tau "/1
  Gain3/1 -> Add1/2
  "u "/1 -> Gain3/1
  Trigonometric Function1/1 -> Product1/1
  q/1 -> Trigonometric Function1/1

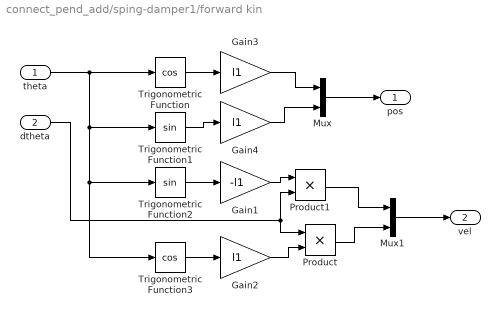
== system connect_pend_add/sping-damper1/forward kin ==
  "theta " : Inport
  "dtheta " : Inport  Port=2
  Gain1 : Gain  Gain=-l1
  Gain2 : Gain  Gain=l1
  Gain3 : Gain  Gain=l1
  Gain4 : Gain  Gain=l1
  Mux : Mux  Inputs=2
  Mux1 : Mux  Inputs=2
  Product : Product
  Product1 : Product
  Trigonometric Function : Trigonometry  Operator=cos
  Trigonometric Function1 : Trigonometry
  Trigonometric Function2 : Trigonometry
  Trigonometric Function3 : Trigonometry  Operator=cos
  pos : Outport
  vel : Outport  Port=2
  wires:
  "theta "/1 -> Trigonometric Function3/1, Trigonometric Function2/1, Trigonometric Function1/1, Trigonometric Function/1
  Gain4/1 -> Mux/2
  Trigonometric Function/1 -> Gain3/1
  Gain3/1 -> Mux/1
  Trigonometric Function1/1 -> Gain4/1
  Trigonometric Function3/1 -> Gain2/1
  Trigonometric Function2/1 -> Gain1/1
  Gain1/1 -> Product1/1
  "dtheta "/1 -> Product1/2, Product/1
  Gain2/1 -> Product/2
  Product1/1 -> Mux1/1
  Product/1 -> Mux1/2
  Mux/1 -> pos/1
  Mux1/1 -> vel/1

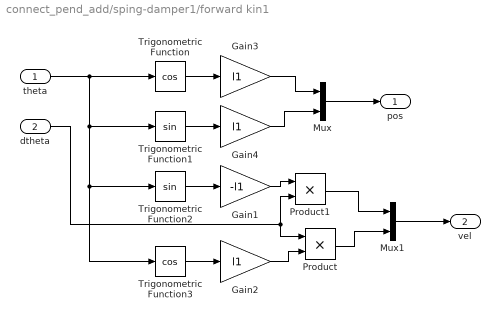
== system connect_pend_add/sping-damper1/forward kin1 ==
  "theta " : Inport
  "dtheta " : Inport  Port=2
  Gain1 : Gain  Gain=-l1
  Gain2 : Gain  Gain=l1
  Gain3 : Gain  Gain=l1
  Gain4 : Gain  Gain=l1
  Mux : Mux  Inputs=2
  Mux1 : Mux  Inputs=2
  Product : Product
  Product1 : Product
  Trigonometric Function : Trigonometry  Operator=cos
  Trigonometric Function1 : Trigonometry
  Trigonometric Function2 : Trigonometry
  Trigonometric Function3 : Trigonometry  Operator=cos
  pos : Outport
  vel : Outport  Port=2
  wires:
  "theta "/1 -> Trigonometric Function3/1, Trigonometric Function2/1, Trigonometric Function1/1, Trigonometric Function/1
  Gain4/1 -> Mux/2
  Trigonometric Function/1 -> Gain3/1
  Gain3/1 -> Mux/1
  Trigonometric Function1/1 -> Gain4/1
  Trigonometric Function3/1 -> Gain2/1
  Trigonometric Function2/1 -> Gain1/1
  Gain1/1 -> Product1/1
  "dtheta "/1 -> Product1/2, Product/1
  Gain2/1 -> Product/2
  Product1/1 -> Mux1/1
  Product/1 -> Mux1/2
  Mux/1 -> pos/1
  Mux1/1 -> vel/1

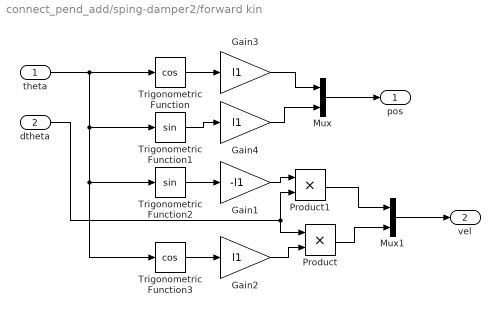
== system connect_pend_add/sping-damper2/forward kin ==
  "theta " : Inport
  "dtheta " : Inport  Port=2
  Gain1 : Gain  Gain=-l1
  Gain2 : Gain  Gain=l1
  Gain3 : Gain  Gain=l1
  Gain4 : Gain  Gain=l1
  Mux : Mux  Inputs=2
  Mux1 : Mux  Inputs=2
  Product : Product
  Product1 : Product
  Trigonometric Function : Trigonometry  Operator=cos
  Trigonometric Function1 : Trigonometry
  Trigonometric Function2 : Trigonometry
  Trigonometric Function3 : Trigonometry  Operator=cos
  pos : Outport
  vel : Outport  Port=2
  wires:
  "theta "/1 -> Trigonometric Function3/1, Trigonometric Function2/1, Trigonometric Function1/1, Trigonometric Function/1
  Gain4/1 -> Mux/2
  Trigonometric Function/1 -> Gain3/1
  Gain3/1 -> Mux/1
  Trigonometric Function1/1 -> Gain4/1
  Trigonometric Function3/1 -> Gain2/1
  Trigonometric Function2/1 -> Gain1/1
  Gain1/1 -> Product1/1
  "dtheta "/1 -> Product1/2, Product/1
  Gain2/1 -> Product/2
  Product1/1 -> Mux1/1
  Product/1 -> Mux1/2
  Mux/1 -> pos/1
  Mux1/1 -> vel/1

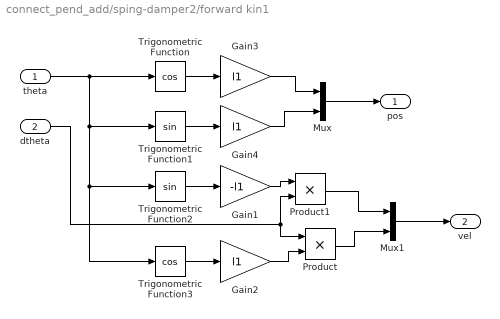
== system connect_pend_add/sping-damper2/forward kin1 ==
  "theta " : Inport
  "dtheta " : Inport  Port=2
  Gain1 : Gain  Gain=-l1
  Gain2 : Gain  Gain=l1
  Gain3 : Gain  Gain=l1
  Gain4 : Gain  Gain=l1
  Mux : Mux  Inputs=2
  Mux1 : Mux  Inputs=2
  Product : Product
  Product1 : Product
  Trigonometric Function : Trigonometry  Operator=cos
  Trigonometric Function1 : Trigonometry
  Trigonometric Function2 : Trigonometry
  Trigonometric Function3 : Trigonometry  Operator=cos
  pos : Outport
  vel : Outport  Port=2
  wires:
  "theta "/1 -> Trigonometric Function3/1, Trigonometric Function2/1, Trigonometric Function1/1, Trigonometric Function/1
  Gain4/1 -> Mux/2
  Trigonometric Function/1 -> Gain3/1
  Gain3/1 -> Mux/1
  Trigonometric Function1/1 -> Gain4/1
  Trigonometric Function3/1 -> Gain2/1
  Trigonometric Function2/1 -> Gain1/1
  Gain1/1 -> Product1/1
  "dtheta "/1 -> Product1/2, Product/1
  Gain2/1 -> Product/2
  Product1/1 -> Mux1/1
  Product/1 -> Mux1/2
  Mux/1 -> pos/1
  Mux1/1 -> vel/1
